simulink library "Vehicle_cl"  (R2020a)
settings: Solver=VariableStepAuto  StartTime=0.0  StopTime=10.0  RelTol=1e-3
undefined symbols (not defined in the file): CFN, EGR, ENG, ENV, ETM, FAN, IC, ICE, magnitude, RAD, TRAN, TSTAT, VEH, x_0
libraries: simulink_extras x2
settings Model: Creator=John Jr  LastModifiedBy=John Jr

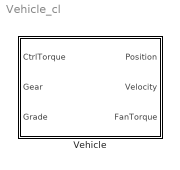
== system Vehicle_cl ==
  Vehicle : Subsystem

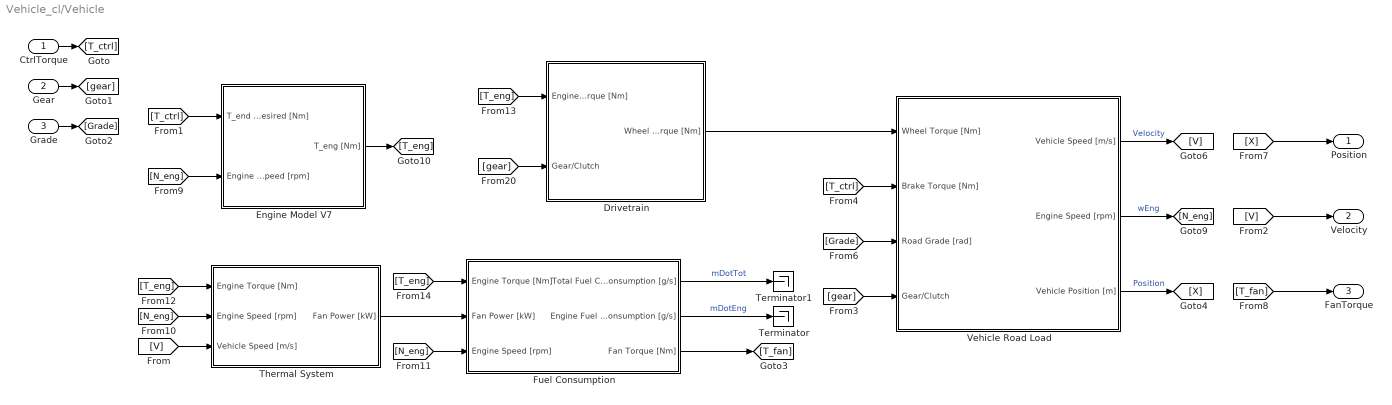
== system Vehicle_cl/Vehicle ==
  CtrlTorque : Inport
  Gear : Inport  Port=2
  Grade : Inport  Port=3
  Drivetrain : Subsystem
  Engine Model V7 : Subsystem
  Fuel Consumption : Subsystem
  Terminator : Terminator
  Terminator1 : Terminator
  Thermal System : Subsystem
  Vehicle Road Load : Subsystem
  Position : Outport
  Velocity : Outport  Port=2
  FanTorque : Outport  Port=3
  wires:
  [T_eng] -> Drivetrain/1(EngineTorque [Nm])
  Fuel Consumption/2(Engine Fuel Consumption [g/s]) -> Terminator/1  "mDotEng"
  [Grade] -> Vehicle Road Load/3(Road Grade [rad])
  [N_eng] -> Fuel Consumption/3(Engine Speed [rpm])
  Vehicle Road Load/3(Vehicle Position [m]) -> [X]  "Position"
  Fuel Consumption/3(Fan Torque [Nm]) -> [T_fan]
  Fuel Consumption/1(Total Fuel Consumption [g/s]) -> Terminator1/1  "mDotTot"
  Gear/1 -> [gear]
  Vehicle Road Load/2(Engine Speed [rpm]) -> [N_eng]  "wEng"
  [T_eng] -> Thermal System/1(Engine Torque [Nm])
  [T_ctrl] -> Vehicle Road Load/2(Brake Torque [Nm])
  [gear] -> Vehicle Road Load/4("Gear/Clutch ")
  [T_eng] -> Fuel Consumption/1(Engine Torque [Nm])
  [T_ctrl] -> Engine Model V7/1(T_end Desired [Nm])
  [gear] -> Drivetrain/2(Gear/Clutch)
  CtrlTorque/1 -> [T_ctrl]
  [N_eng] -> Engine Model V7/2(Engine Speed [rpm])
  Engine Model V7/1(T_eng [Nm]) -> [T_eng]
  [V] -> Thermal System/3(Vehicle Speed [m/s])
  Vehicle Road Load/1(Vehicle Speed [m/s]) -> [V]  "Velocity"
  Drivetrain/1(Wheel Torque [Nm]) -> Vehicle Road Load/1(Wheel Torque [Nm])
  [N_eng] -> Thermal System/2(Engine Speed [rpm])
  Thermal System/1(" Fan Power [kW]") -> Fuel Consumption/2(" Fan Power [kW]")
  Grade/1 -> [Grade]
  [T_fan] -> FanTorque/1
  [V] -> Velocity/1
  [X] -> Position/1

== system Vehicle_cl/Vehicle/Drivetrain ==
  EngineTorque [Nm] : Inport
  Gear/Clutch : Inport  Port=2
  Bus Selector : BusSelector  OutputSignals=Gear
  Gain2 : Gain  Gain=TRAN.finalDrive
  Gain3 : Gain  Gain=TRAN.gearEfficiency
  Gear Ratios : Lookup_n-D  NumberOfTableDimensions=1  BreakpointsForDimension1=[1:TRAN.numGears]  Table=TRAN.gears  ExtrapMethod=Clip  UseLastTableValue=on  InternalRulePriority=Speed  RndMeth=Simplest  InputSameDT=on
  Product1 : Product  Inputs=3
  Round : Rounding  Operator=round
  Transfe Fcn (with initial outputs) : simulink_extras/Additional Linear/Transfer Fcn (with initial outputs)  N=[1]  D="[.04 .4  1]"  Y0=0  U0=0
  Transmission Efficiency : Lookup_n-D  NumberOfTableDimensions=1  BreakpointsForDimension1=[1:TRAN.numGears]  Table=TRAN.transEfficiency  ExtrapMethod=Clip  UseLastTableValue=on  InternalRulePriority=Speed  RndMeth=Simplest  InputSameDT=on
  Wheel Torque [Nm] : Outport  VectorParamsAs1DForOutWhenUnconnected=off
  wires:
  Gear Ratios/1 -> Gain2/1
  Gain2/1 -> Product1/3
  Transmission Efficiency/1 -> Gain3/1
  Gain3/1 -> Product1/2
  Product1/1 -> Wheel Torque [Nm]/1  "whlTorque"
  EngineTorque [Nm]/1 -> Product1/1
  Transfe Fcn (with initial outputs)/1 -> Transmission Efficiency/1, Round/1
  Gear/Clutch/1 -> Bus Selector/1
  Bus Selector/1 -> Transfe Fcn (with initial outputs)/1  "<Gear>"
  Round/1 -> Gear Ratios/1

== system Vehicle_cl/Vehicle/Engine Model V7 ==
  T_end Desired [Nm] : Inport
  Engine Speed [rpm] : Inport  Port=2
  Bus Selector : BusSelector  OutputSignals=T_eng
  "Engine Breathing " : Subsystem
  Fuel Model : Subsystem
  Torque Production : Subsystem
  T_eng [Nm] : Outport  VectorParamsAs1DForOutWhenUnconnected=off
  wires:
  "Engine Breathing "/1(m_eng [kg/s]) -> Fuel Model/2(m_dot_eng [kg/s])
  Fuel Model/1(fuel [mg/cyc]) -> Torque Production/2(fuel [mg/cyc])
  Engine Speed [rpm]/1 -> "Engine Breathing "/1(Engine Speed [rpm]), Fuel Model/1(N [RPM]), Torque Production/1(N [RPM])
  Torque Production/1(T_eng [Nm]) -> T_eng [Nm]/1  "T_eng_act"
  T_end Desired [Nm]/1 -> Bus Selector/1
  Bus Selector/1 -> Torque Production/3(Engine Torqe Des [Nm]), Fuel Model/3(Engine Torqe Des [Nm]), "Engine Breathing "/2(Engine Torqe Des [Nm])  "<T_eng>"

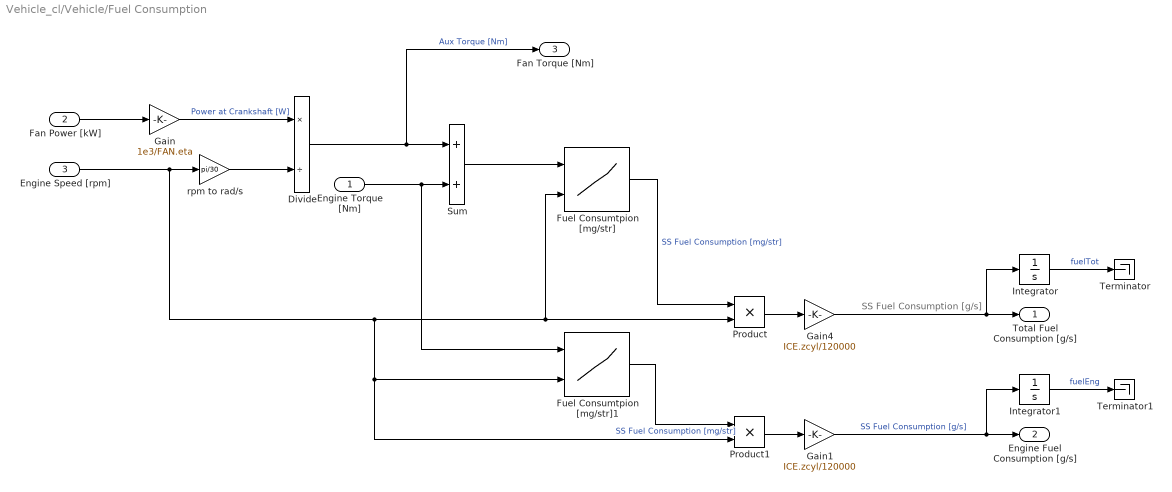
== system Vehicle_cl/Vehicle/Fuel Consumption ==
  note: SS Fuel Consumption [g/s]
  Engine Torque [Nm] : Inport
  " Fan Power [kW]" : Inport  Port=2
  Engine Speed [rpm] : Inport  Port=3
  Divide : Product  Inputs=*/
  Fuel Consumtpion [mg/str] : Lookup_n-D  BreakpointsForDimension1=ICE.FC.T  BreakpointsForDimension2=ICE.FC.N  Table=ICE.FC.mdot_mgpstr  InternalRulePriority=Speed  RndMeth=Simplest  InputSameDT=on
  Fuel Consumtpion [mg/str]1 : Lookup_n-D  BreakpointsForDimension1=ICE.FC.T  BreakpointsForDimension2=ICE.FC.N  Table=ICE.FC.mdot_mgpstr  InternalRulePriority=Speed  RndMeth=Simplest  InputSameDT=on
  Gain : Gain  Gain=1e3/FAN.eta
  Gain1 : Gain  Gain=ICE.zcyl/120000
  Gain4 : Gain  Gain=ICE.zcyl/120000
  Integrator : Integrator
  Integrator1 : Integrator
  Product : Product
  Product1 : Product
  Sum : Sum
  Terminator : Terminator
  Terminator1 : Terminator
  rpm to rad/s : Gain  Gain=pi/30
  Total Fuel Consumption [g/s] : Outport  VectorParamsAs1DForOutWhenUnconnected=off
  Engine Fuel Consumption [g/s] : Outport  Port=2  VectorParamsAs1DForOutWhenUnconnected=off
  Fan Torque [Nm] : Outport  Port=3  VectorParamsAs1DForOutWhenUnconnected=off
  wires:
  " Fan Power [kW]"/1 -> Gain/1
  Gain/1 -> Divide/1  "Power at Crankshaft [W]"
  rpm to rad/s/1 -> Divide/2
  Divide/1 -> Fan Torque [Nm]/1, Sum/1  "Aux Torque [Nm]"
  Gain4/1 -> Integrator/1, Total Fuel Consumption [g/s]/1
  Gain1/1 -> Integrator1/1, Engine Fuel Consumption [g/s]/1  "SS Fuel Consumption [g/s]"
  Fuel Consumtpion [mg/str]/1 -> Product/1  "SS Fuel Consumption [mg/str]"
  Product/1 -> Gain4/1
  Sum/1 -> Fuel Consumtpion [mg/str]/1
  Engine Speed [rpm]/1 -> Product1/2, Fuel Consumtpion [mg/str]1/2, Fuel Consumtpion [mg/str]/2, Product/2, rpm to rad/s/1
  Fuel Consumtpion [mg/str]1/1 -> Product1/1  "SS Fuel Consumption [mg/str]"
  Product1/1 -> Gain1/1
  Engine Torque [Nm]/1 -> Fuel Consumtpion [mg/str]1/1, Sum/2
  Integrator/1 -> Terminator/1  "fuelTot"
  Integrator1/1 -> Terminator1/1  "fuelEng"

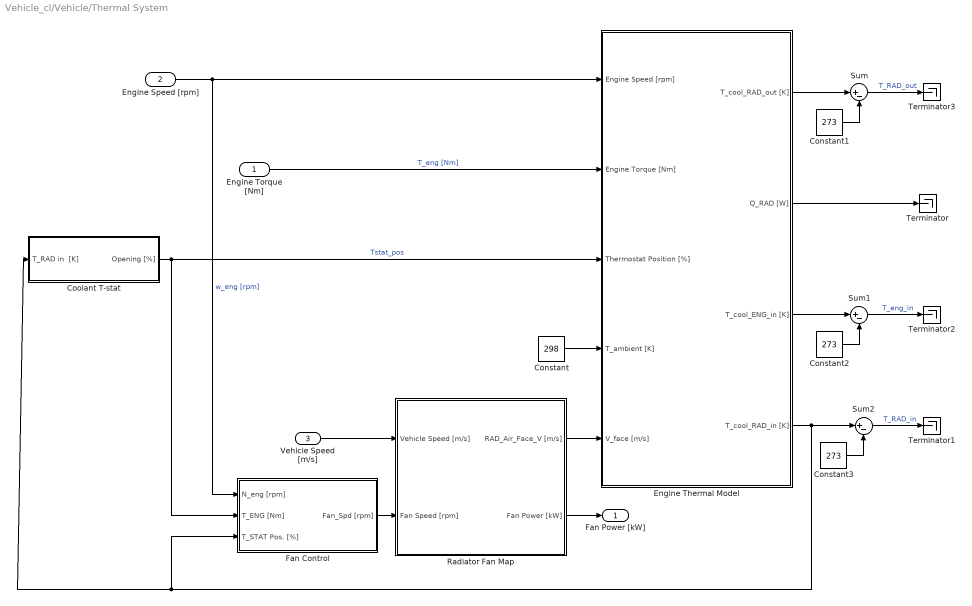
== system Vehicle_cl/Vehicle/Thermal System ==
  Engine Torque [Nm] : Inport
  Engine Speed [rpm] : Inport  Port=2
  Vehicle Speed [m/s] : Inport  Port=3
  Constant : Constant  Value=298
  Constant1 : Constant  Value=273
  Constant2 : Constant  Value=273
  Constant3 : Constant  Value=273
  Coolant T-stat : Subsystem
  Engine Thermal Model : Subsystem
  Fan Control : Subsystem
  Radiator Fan Map : Subsystem
  Sum : Sum  Inputs=|+-
  Sum1 : Sum  Inputs=|+-
  Sum2 : Sum  Inputs=|+-
  Terminator{,1..3} (4 alike) : Terminator
  " Fan Power [kW]" : Outport  VectorParamsAs1DForOutWhenUnconnected=off
  wires:
  Fan Control/1(Fan_Spd [rpm]) -> Radiator Fan Map/2(Fan Speed [rpm])
  Engine Speed [rpm]/1 -> Fan Control/1(N_eng [rpm]), Engine Thermal Model/1(Engine Speed [rpm])  "w_eng [rpm]"
  Radiator Fan Map/2(Fan Power [kW]) -> " Fan Power [kW]"/1
  Constant/1 -> Engine Thermal Model/4(T_ambient [K])
  Engine Torque [Nm]/1 -> Engine Thermal Model/2(Engine Torque [Nm])  "T_eng [Nm]"
  Radiator Fan Map/1(RAD_Air_Face_V [m/s]) -> Engine Thermal Model/5(V_face [m/s])
  Engine Thermal Model/1(T_cool_RAD_out [K]) -> Sum/1
  Constant1/1 -> Sum/2
  Sum/1 -> Terminator3/1  "T_RAD_out"
  Engine Thermal Model/3(T_cool_ENG_in [K]) -> Sum1/1
  Constant2/1 -> Sum1/2
  Sum1/1 -> Terminator2/1  "T_eng_in"
  Engine Thermal Model/4(T_cool_RAD_in [K]) -> Sum2/1, Fan Control/3(T_STAT Pos. [%]), Coolant T-stat/1(T_RAD in  [K])
  Constant3/1 -> Sum2/2
  Sum2/1 -> Terminator1/1  "T_RAD_in"
  Vehicle Speed [m/s]/1 -> Radiator Fan Map/1(Vehicle Speed [m/s])
  Engine Thermal Model/2(Q_RAD [W]) -> Terminator/1
  Coolant T-stat/1(Opening [%]) -> Fan Control/2(T_ENG [Nm]), Engine Thermal Model/3(Thermostat Position [%])  "Tstat_pos"

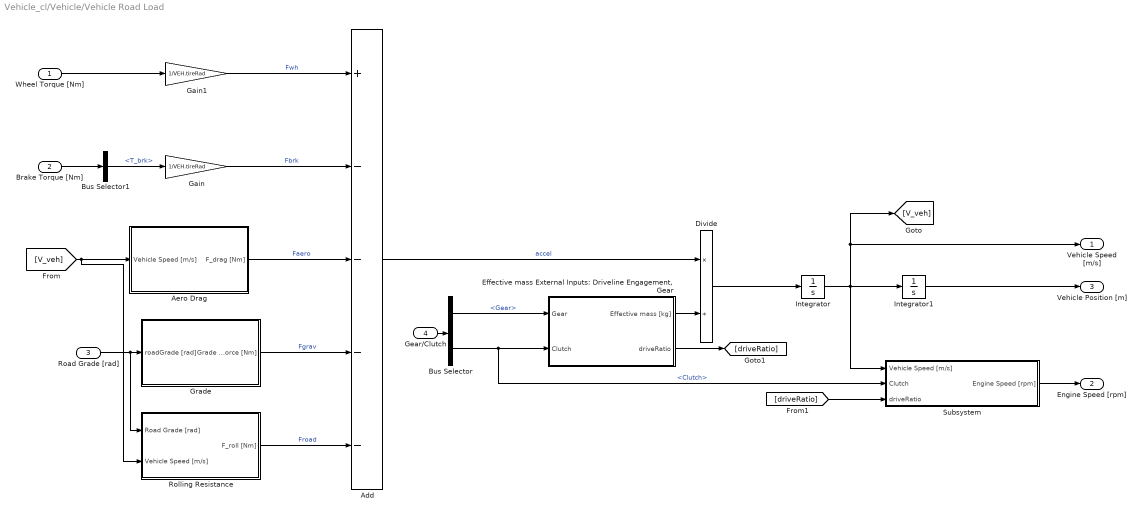
== system Vehicle_cl/Vehicle/Vehicle Road Load ==
  Wheel Torque [Nm] : Inport
  Brake Torque [Nm] : Inport  Port=2
  Road Grade [rad] : Inport  Port=3
  "Gear/Clutch " : Inport  Port=4
  Add : Sum  Inputs=+----
  Aero Drag : Subsystem
  Bus Selector : BusSelector  OutputSignals=Gear,Clutch
  Bus Selector1 : BusSelector  OutputSignals=T_brk
  Divide : Product  Inputs=*/
  "Effective mass External Inputs: Driveline Engagement, Gear" : Subsystem
  Gain : Gain  Gain=1/VEH.tireRad
  Gain1 : Gain  Gain=1/VEH.tireRad
  Grade : Subsystem
  Integrator : Integrator  LimitOutput=on  LowerSaturationLimit=0
  Integrator1 : Integrator  InitialCondition=x_0  LimitOutput=on  LowerSaturationLimit=0
  Rolling Resistance : Subsystem
  Subsystem : Subsystem
  Vehicle Speed [m/s] : Outport  VectorParamsAs1DForOutWhenUnconnected=off
  Engine Speed [rpm] : Outport  Port=2  VectorParamsAs1DForOutWhenUnconnected=off
  Vehicle Position [m] : Outport  Port=3  VectorParamsAs1DForOutWhenUnconnected=off
  wires:
  Integrator/1 -> Subsystem/1(Vehicle Speed [m/s]), Integrator1/1, Vehicle Speed [m/s]/1, [V_veh]
  Aero Drag/1(F_drag [Nm]) -> Add/3  "Faero"
  Grade/1(Grade Force [Nm]) -> Add/4  "Fgrav"
  Gain/1 -> Add/2  "Fbrk"
  Wheel Torque [Nm]/1 -> Gain1/1
  Gain1/1 -> Add/1  "Fwh"
  Rolling Resistance/1(F_roll [Nm]) -> Add/5  "Froad"
  Add/1 -> Divide/1  "accel"
  Divide/1 -> Integrator/1
  [V_veh] -> Aero Drag/1(Vehicle Speed [m/s]), Rolling Resistance/2(Vehicle Speed [m/s])
  Road Grade [rad]/1 -> Rolling Resistance/1(Road Grade [rad]), Grade/1(roadGrade [rad])
  Subsystem/1(Engine Speed [rpm]) -> Engine Speed [rpm]/1
  "Effective mass External Inputs: Driveline Engagement, Gear"/1("Effective mass [kg] ") -> Divide/2
  Integrator1/1 -> Vehicle Position [m]/1
  "Gear/Clutch "/1 -> Bus Selector/1
  Bus Selector/1 -> "Effective mass External Inputs: Driveline Engagement, Gear"/1(Gear)  "<Gear>"
  Bus Selector/2 -> Subsystem/2(Clutch), "Effective mass External Inputs: Driveline Engagement, Gear"/2(Clutch)  "<Clutch>"
  Brake Torque [Nm]/1 -> Bus Selector1/1
  Bus Selector1/1 -> Gain/1  "<T_brk>"
  "Effective mass External Inputs: Driveline Engagement, Gear"/2(driveRatio) -> [driveRatio]
  [driveRatio] -> Subsystem/3(driveRatio)

== system Vehicle_cl/Vehicle/Engine Model V7/Engine Breathing  ==
  Engine Speed [rpm] : Inport
  Engine Torqe Des [Nm] : Inport  Port=2
  Air Dynamics : Subsystem
  Engine Torqe Des [Nm]1 : InportShadow  Port=2
  Gain : Gain  Gain=1e3
  Gain1 : Gain  Gain=ICE.Vd/(120*ENV.R)
  Intake Manifold Pressure [kPa] : Lookup_n-D  BreakpointsForDimension1=ICE.air.Torque  BreakpointsForDimension2=ICE.air.N  Table=ICE.air.MAP  InternalRulePriority=Speed  RndMeth=Simplest  InputSameDT=on
  Intake Manifold Temperature [K] : Lookup_n-D  BreakpointsForDimension1=ICE.air.Torque  BreakpointsForDimension2=ICE.air.N  Table=ICE.air.MAT  InternalRulePriority=Speed  RndMeth=Simplest  InputSameDT=on
  Memory : Memory
  Model for VE : Subsystem
  Product : Product  Inputs=***/
  Subtract : Sum  Inputs=+-
  m_eng [kg/s] : Outport  VectorParamsAs1DForOutWhenUnconnected=off
  wires:
  Model for VE/1(VE [-]) -> Product/1
  Product/1 -> Gain1/1
  Gain1/1 -> Air Dynamics/1(m_dot_SS [kg/s])  "m_dot_SS"
  Intake Manifold Temperature [K]/1 -> Product/4, Model for VE/2(TIM [K])
  Engine Speed [rpm]/1 -> Intake Manifold Pressure [kPa]/2, Intake Manifold Temperature [K]/2, Product/3, Model for VE/3(N_eng [RPM])
  Engine Torqe Des [Nm]/1 -> Intake Manifold Temperature [K]/1, Intake Manifold Pressure [kPa]/1
  Gain/1 -> Product/2
  Intake Manifold Pressure [kPa]/1 -> Gain/1, Model for VE/1(MAP [kPa])
  Air Dynamics/1(m_dot_eng [kg/s]) -> m_eng [kg/s]/1  "m_dot_eng"
  Engine Torqe Des [Nm]1/1 -> Memory/1, Subtract/1
  Memory/1 -> Subtract/2
  Subtract/1 -> Air Dynamics/2(detla Torque [Nm])  "\\delta T Requested"

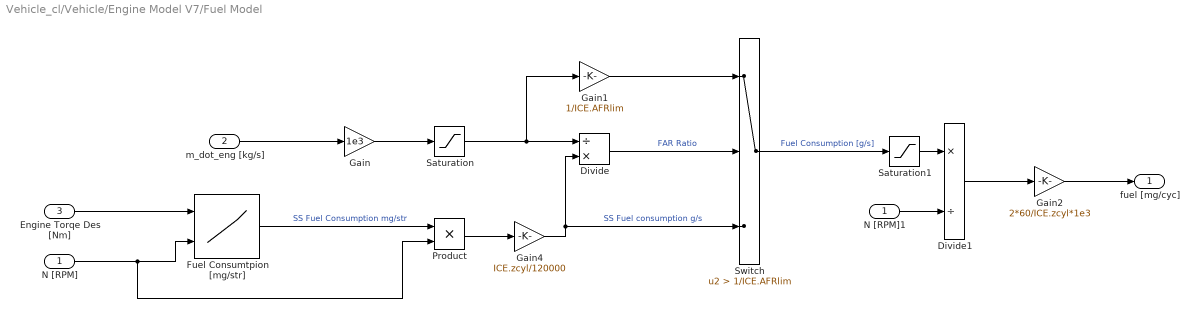
== system Vehicle_cl/Vehicle/Engine Model V7/Fuel Model ==
  N [RPM] : Inport
  m_dot_eng [kg/s] : Inport  Port=2
  Engine Torqe Des [Nm] : Inport  Port=3
  Divide : Product  Inputs=/*
  Divide1 : Product  Inputs=*/
  Fuel Consumtpion [mg/str] : Lookup_n-D  BreakpointsForDimension1=ICE.FC.T  BreakpointsForDimension2=ICE.FC.N  Table=ICE.FC.mdot_mgpstr  InternalRulePriority=Speed  RndMeth=Simplest  InputSameDT=on
  Gain : Gain  Gain=1e3
  Gain1 : Gain  Gain=1/ICE.AFRlim
  Gain2 : Gain  Gain=2*60/ICE.zcyl*1e3
  Gain4 : Gain  Gain=ICE.zcyl/120000
  N [RPM]1 : InportShadow
  Product : Product
  Saturation : Saturate  UpperLimit=inf  LowerLimit=0.001
  Saturation1 : Saturate  UpperLimit=inf  LowerLimit=0
  Switch : Switch  Criteria=u2 > Threshold  Threshold=1/ICE.AFRlim
  fuel [mg/cyc] : Outport  VectorParamsAs1DForOutWhenUnconnected=off
  wires:
  m_dot_eng [kg/s]/1 -> Gain/1
  N [RPM]/1 -> Product/2, Fuel Consumtpion [mg/str]/2
  Divide/1 -> Switch/2  "FAR Ratio"
  Fuel Consumtpion [mg/str]/1 -> Product/1  "SS Fuel Consumption mg/str"
  Gain/1 -> Saturation/1
  Gain1/1 -> Switch/1
  N [RPM]1/1 -> Divide1/2
  Divide1/1 -> Gain2/1
  Switch/1 -> Saturation1/1  "Fuel Consumption [g/s]"
  Saturation/1 -> Gain1/1, Divide/1
  Gain2/1 -> fuel [mg/cyc]/1
  Saturation1/1 -> Divide1/1
  Product/1 -> Gain4/1
  Gain4/1 -> Switch/3, Divide/2  "SS Fuel consumption g/s"
  Engine Torqe Des [Nm]/1 -> Fuel Consumtpion [mg/str]/1

== system Vehicle_cl/Vehicle/Engine Model V7/Torque Production ==
  N [RPM] : Inport
  fuel [mg/cyc] : Inport  Port=2
  Engine Torqe Des [Nm] : Inport  Port=3
  Add : Sum  Inputs=+--
  Constant : Constant  Value=0
  Constant1 : Constant  Value=40/ICE.Vd*(4*pi)
  FMEP Model : Lookup_n-D  BreakpointsForDimension1=ICE.FMEP.RPM_vec  BreakpointsForDimension2=ICE.FMEP.fuel_vec  Table=ICE.FMEP.FMEP_surf  InternalRulePriority=Speed  RndMeth=Simplest  InputSameDT=on
  Fuel Dynamics : Subsystem
  Gain1 : Gain  Gain=ICE.Vd/(4*pi)
  IMEP Model : Lookup_n-D  BreakpointsForDimension1=ICE.IMEP.N  BreakpointsForDimension2=ICE.IMEP.m_fuel  Table=ICE.IMEP.IMEP'  UseLastTableValue=on  InternalRulePriority=Speed  RndMeth=Simplest  InputSameDT=on
  Memory : Memory
  Subtract : Sum  Inputs=+-
  Switch : Switch  Criteria=u2 > Threshold
  T_eng [Nm] : Outport  VectorParamsAs1DForOutWhenUnconnected=off
  wires:
  FMEP Model/1 -> Add/2  "FMEP [Pa]"
  IMEP Model/1 -> Add/1  "IMEP [Pa]"
  Add/1 -> Gain1/1  "BMEP [Pa]"
  N [RPM]/1 -> IMEP Model/1, FMEP Model/1
  fuel [mg/cyc]/1 -> IMEP Model/2, Switch/2, FMEP Model/2
  Gain1/1 -> Fuel Dynamics/1(T_SS [Nm])
  Engine Torqe Des [Nm]/1 -> Memory/1, Subtract/1
  Memory/1 -> Subtract/2
  Subtract/1 -> Fuel Dynamics/2(detla Torque [Nm])  "\\delta T Requested"
  Fuel Dynamics/1(Torque [Nm]) -> T_eng [Nm]/1
  Switch/1 -> Add/3
  Constant/1 -> Switch/1
  Constant1/1 -> Switch/3

== system Vehicle_cl/Vehicle/Thermal System/Coolant T-stat ==
  T_RAD in  [K] : Inport
  Add : Sum
  Constant : Constant  Value=TSTAT.tau
  Divide : Product  Inputs=*/
  Fcn1 : Fcn  Expr=u-273
  Gain : Gain  Gain=0.85
  Gain1 : Gain  Gain=0.15
  Integrator : Integrator  InitialCondition=TSTAT.IC
  Sum : Sum  Inputs=+-
  Temp - Mechanical Closing : Lookup  InputValues=TSTAT.mclosing(:,1)  Table=TSTAT.mclosing(:,2)  LookUpMeth=Interpolation-Use End Values
  Temp - Mechanical Opening : Lookup  InputValues=TSTAT.mopening(:,1)  Table=TSTAT.mopening(:,2)  LookUpMeth=Interpolation-Use End Values
  Opening [%] : Outport  VectorParamsAs1DForOutWhenUnconnected=off
  wires:
  Temp - Mechanical Opening/1 -> Gain/1
  Temp - Mechanical Closing/1 -> Gain1/1
  Add/1 -> Sum/1
  Sum/1 -> Divide/1
  Constant/1 -> Divide/2
  Divide/1 -> Integrator/1
  Integrator/1 -> Sum/2, Opening [%]/1
  T_RAD in  [K]/1 -> Fcn1/1
  Gain/1 -> Add/1
  Gain1/1 -> Add/2
  Fcn1/1 -> Temp - Mechanical Opening/1, Temp - Mechanical Closing/1

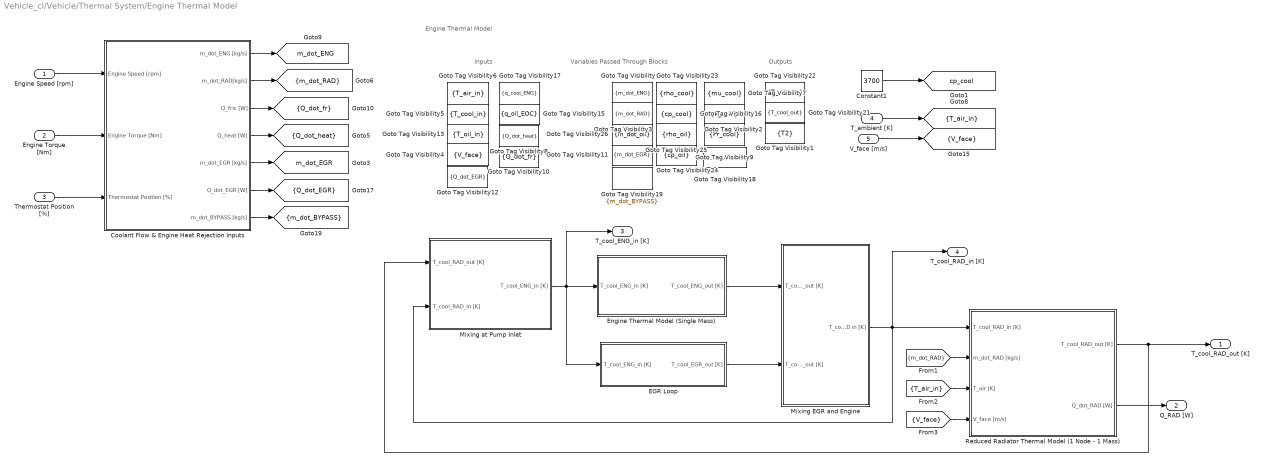
== system Vehicle_cl/Vehicle/Thermal System/Engine Thermal Model ==
  note: Variables Passed Through Blocks
  note: Inputs
  note: Engine Thermal Model
  note: Outputs
  Engine Speed [rpm] : Inport
  Engine Torque [Nm] : Inport  Port=2
  Thermostat Position [%] : Inport  Port=3
  T_ambient [K] : Inport  Port=4
  V_face [m/s] : Inport  Port=5
  Constant1 : Constant  Value=3700
  Coolant Flow & Engine Heat Rejection Inputs : Subsystem
      mask DialogControl DescGroupVar Prompt: Coolant Flow Rate And Engine Heat Rejection Inputs
  EGR Loop : Subsystem
  Engine Thermal Model (Single Mass) : Subsystem
  Goto Tag Visibility1 : GotoTagVisibility  GotoTag=T2
  Goto Tag Visibility10 : GotoTagVisibility  GotoTag=Q_dot_fr
  Goto Tag Visibility11 : GotoTagVisibility  GotoTag=m_dot_EGR
  Goto Tag Visibility12 : GotoTagVisibility  GotoTag=Q_dot_EGR
  Goto Tag Visibility13 : GotoTagVisibility  GotoTag=T_oil_in
  Goto Tag Visibility14 : GotoTagVisibility  GotoTag=m_dot_ENG
  Goto Tag Visibility15 : GotoTagVisibility  GotoTag=q_oil_EOC
  Goto Tag Visibility16 : GotoTagVisibility  GotoTag=cp_cool
  Goto Tag Visibility17 : GotoTagVisibility  GotoTag=q_cool_ENG
  Goto Tag Visibility18 : GotoTagVisibility  GotoTag=T_cool_ENG_out
  Goto Tag Visibility19 : GotoTagVisibility  GotoTag=m_dot_BYPASS
  Goto Tag Visibility2 : GotoTagVisibility  GotoTag=k_cool
  Goto Tag Visibility21 : GotoTagVisibility  GotoTag=T_cool_out
  Goto Tag Visibility22 : GotoTagVisibility  GotoTag=T_oil_out
  Goto Tag Visibility23 : GotoTagVisibility  GotoTag=rho_cool
  Goto Tag Visibility24 : GotoTagVisibility  GotoTag=cp_oil
  Goto Tag Visibility25 : GotoTagVisibility  GotoTag=rho_oil
  Goto Tag Visibility26 : GotoTagVisibility  GotoTag=m_dot_oil
  Goto Tag Visibility3 : GotoTagVisibility  GotoTag=m_dot_RAD
  Goto Tag Visibility4 : GotoTagVisibility  GotoTag=V_face
  Goto Tag Visibility5 : GotoTagVisibility  GotoTag=T_cool_in
  Goto Tag Visibility6 : GotoTagVisibility  GotoTag=T_air_in
  Goto Tag Visibility7 : GotoTagVisibility  GotoTag=mu_cool
  Goto Tag Visibility8 : GotoTagVisibility  GotoTag=Q_dot_heat
  Goto Tag Visibility9 : GotoTagVisibility  GotoTag=Pr_cool
  Mixing EGR and Engine : Subsystem
  "Mixing at Pump Inlet " : Subsystem
  Reduced Radiator Thermal Model (1 Node - 1 Mass) : Subsystem
  T_cool_RAD_out [K] : Outport  VectorParamsAs1DForOutWhenUnconnected=off
  Q_RAD [W] : Outport  Port=2  VectorParamsAs1DForOutWhenUnconnected=off
  T_cool_ENG_in [K] : Outport  Port=3  VectorParamsAs1DForOutWhenUnconnected=off
  T_cool_RAD_in [K] : Outport  Port=4  VectorParamsAs1DForOutWhenUnconnected=off
  tag scope: Q_dot_EGR=scoped, Q_dot_fr=scoped, Q_dot_heat=scoped, T_air_in=scoped, V_face=scoped, cp_cool=global, m_dot_BYPASS=scoped, m_dot_EGR=global, m_dot_ENG=global, m_dot_RAD=scoped
  wires:
  T_ambient [K]/1 -> [T_air_in]
  [m_dot_RAD] -> Reduced Radiator Thermal Model (1 Node - 1 Mass)/2(m_dot_RAD [kg/s])
  [T_air_in] -> Reduced Radiator Thermal Model (1 Node - 1 Mass)/3(T_air [K])
  V_face [m/s]/1 -> [V_face]
  [V_face] -> Reduced Radiator Thermal Model (1 Node - 1 Mass)/4(V_face [m/s])
  Reduced Radiator Thermal Model (1 Node - 1 Mass)/2(Q_dot_RAD [W]) -> Q_RAD [W]/1
  Reduced Radiator Thermal Model (1 Node - 1 Mass)/1(T_cool_RAD_out [K]) -> "Mixing at Pump Inlet "/1(T_cool_RAD_out [K]), T_cool_RAD_out [K]/1
  Constant1/1 -> [cp_cool]
  Coolant Flow & Engine Heat Rejection Inputs/5(m_dot_EGR [kg/s]) -> [m_dot_EGR]
  Coolant Flow & Engine Heat Rejection Inputs/6(Q_dot_EGR [W]) -> [Q_dot_EGR]
  Coolant Flow & Engine Heat Rejection Inputs/1(m_dot_ENG [kg/s]) -> [m_dot_ENG]
  Coolant Flow & Engine Heat Rejection Inputs/4(Q_heat [W]) -> [Q_dot_heat]
  Coolant Flow & Engine Heat Rejection Inputs/2(m_dot_RAD[kg/s]) -> [m_dot_RAD]
  Engine Torque [Nm]/1 -> Coolant Flow & Engine Heat Rejection Inputs/2(Engine Torque [Nm])
  Coolant Flow & Engine Heat Rejection Inputs/3(Q_fric [W]) -> [Q_dot_fr]
  Thermostat Position [%]/1 -> Coolant Flow & Engine Heat Rejection Inputs/3(Thermostat Position [%])
  Coolant Flow & Engine Heat Rejection Inputs/7(m_dot_BYPASS [kg/s]) -> [m_dot_BYPASS]
  Engine Speed [rpm]/1 -> Coolant Flow & Engine Heat Rejection Inputs/1(Engine Speed [rpm])
  Engine Thermal Model (Single Mass)/1(T_cool_ENG_out [K]) -> Mixing EGR and Engine/1(T_cool_ENG_out [K])
  EGR Loop/1(T_cool_EGR_out [K]) -> Mixing EGR and Engine/2(T_cool_EGR_out [K])
  Mixing EGR and Engine/1(T_cool_RAD in [K]) -> "Mixing at Pump Inlet "/2(T_cool_RAD_in [K]), Reduced Radiator Thermal Model (1 Node - 1 Mass)/1(T_cool_RAD_in [K]), T_cool_RAD_in [K]/1
  "Mixing at Pump Inlet "/1(T_cool_ENG_in [K]) -> T_cool_ENG_in [K]/1, Engine Thermal Model (Single Mass)/1(T_cool_ENG_in [K]), EGR Loop/1(T_cool_ENG_in [K])

== system Vehicle_cl/Vehicle/Thermal System/Fan Control ==
  note: Fan Controller
  N_eng [rpm] : Inport
  T_ENG [Nm] : Inport  Port=2
  T_STAT Pos. [%] : Inport  Port=3
  Fan Min Speed [rpm] : Constant  Value=200
  Fan OFF : Constant  Value=0
  "Fan ON " : Constant
  Fan Pulley Ratio : Constant  Value=FAN.pulley_ratio
  "IF T_eng is > 367 K and T_stat = 100% open, then Fan ON1" : Switch  Threshold=1
  Logical Operator1 : Logic  AllPortsSameDT=off  OutDataTypeStr=boolean
  Product2 : Product  Inputs=3
  Relay2 : Relay  OnSwitchValue=5  OffSwitchValue=0  OnOutputValue=0  OffOutputValue=1
  Relay3 : Relay  OnSwitchValue=25  OffSwitchValue=20
  Switch1 : Switch  Criteria=u2 > Threshold
  Fan_Spd [rpm] : Outport  VectorParamsAs1DForOutWhenUnconnected=off
  wires:
  Product2/1 -> Switch1/1, Switch1/2
  Relay2/1 -> Logical Operator1/2
  Fan Pulley Ratio/1 -> Product2/1
  T_STAT Pos. [%]/1 -> Relay3/1
  N_eng [rpm]/1 -> Product2/3
  Fan Min Speed [rpm]/1 -> Switch1/3
  Relay3/1 -> Logical Operator1/1
  Logical Operator1/1 -> "IF T_eng is > 367 K and T_stat = 100% open, then Fan ON1"/2
  T_ENG [Nm]/1 -> Relay2/1
  Fan OFF/1 -> "IF T_eng is > 367 K and T_stat = 100% open, then Fan ON1"/3
  "IF T_eng is > 367 K and T_stat = 100% open, then Fan ON1"/1 -> Product2/2
  "Fan ON "/1 -> "IF T_eng is > 367 K and T_stat = 100% open, then Fan ON1"/1
  Switch1/1 -> Fan_Spd [rpm]/1  "fanSpeed"

== system Vehicle_cl/Vehicle/Thermal System/Radiator Fan Map ==
  Vehicle Speed [m/s] : Inport
  Fan Speed [rpm] : Inport  Port=2
  Air Density : Constant  Value=RAD.Air_rho
  Divide : Product  Inputs=*//
  Face Area [m^2] : Constant  Value=RAD.A_face
  Fan Power Consumption [kW] : Lookup_n-D  NumberOfTableDimensions=1  BreakpointsForDimension1=FAN.Speed  Table=FAN.Power  RndMeth=Simplest  InputSameDT=on
  Fan Table : Lookup_n-D  BreakpointsForDimension1=FAN.N  BreakpointsForDimension2=FAN.Vspd  Table=FAN.RAD_AGS_o  ExtrapMethod=Clip  RndMeth=Simplest  InputSameDT=on
  RAD_Air_Face_V [m/s] : Outport  VectorParamsAs1DForOutWhenUnconnected=off
  Fan Power [kW] : Outport  Port=2  VectorParamsAs1DForOutWhenUnconnected=off
  wires:
  Fan Speed [rpm]/1 -> Fan Table/1, Fan Power Consumption [kW]/1
  Fan Table/1 -> Divide/1  "Rad_Air_Face_mdot [kg/s]"
  Divide/1 -> RAD_Air_Face_V [m/s]/1
  Air Density/1 -> Divide/3
  Vehicle Speed [m/s]/1 -> Fan Table/2
  Face Area [m^2]/1 -> Divide/2
  Fan Power Consumption [kW]/1 -> Fan Power [kW]/1

== system Vehicle_cl/Vehicle/Vehicle Road Load/Aero Drag ==
  Vehicle Speed [m/s] : Inport
  Gain1 : Gain  Gain=0.5*VEH.Af*ENV.rhoAir
  Math Function : Math  Operator=magnitude^2  SignedPower=on  SaturateOnIntegerOverflow=on
  Product : Product
  air drag coefficient3 : Constant  Value=VEH.Cd
  F_drag [Nm] : Outport  VectorParamsAs1DForOutWhenUnconnected=off
  wires:
  Vehicle Speed [m/s]/1 -> Math Function/1
  Gain1/1 -> F_drag [Nm]/1  "Drag"
  Math Function/1 -> Product/1
  air drag coefficient3/1 -> Product/2
  Product/1 -> Gain1/1

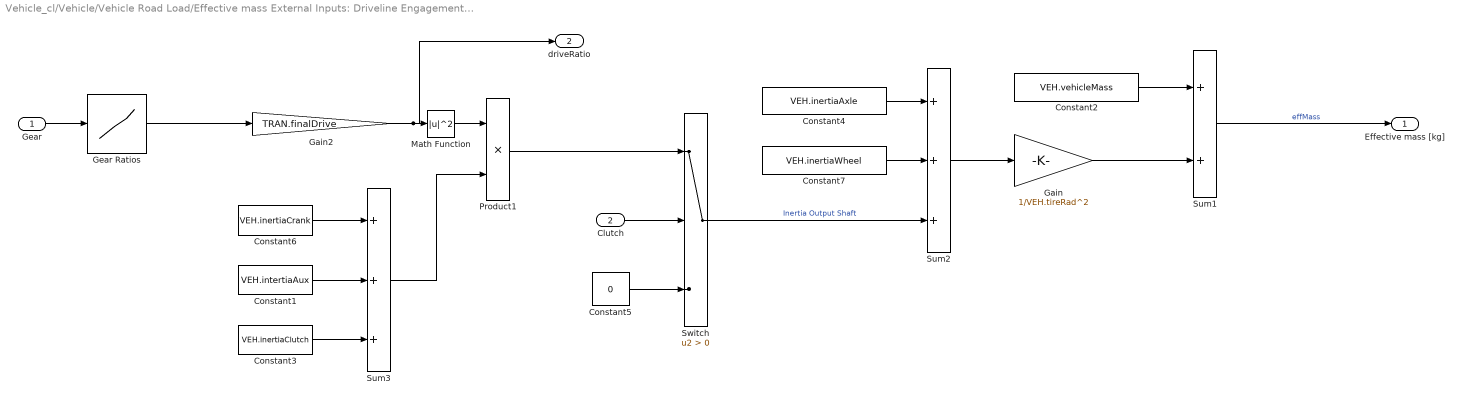
== system Vehicle_cl/Vehicle/Vehicle Road Load/Effective mass External Inputs: Driveline Engagement, Gear ==
  Gear : Inport
  Clutch : Inport  Port=2
  Constant1 : Constant  Value=VEH.intertiaAux
  Constant2 : Constant  Value=VEH.vehicleMass
  Constant3 : Constant  Value=VEH.inertiaClutch
  Constant4 : Constant  Value=VEH.inertiaAxle
  Constant5 : Constant  Value=0
  Constant6 : Constant  Value=VEH.inertiaCrank
  Constant7 : Constant  Value=VEH.inertiaWheel
  Gain : Gain  Gain=1/VEH.tireRad^2
  Gain2 : Gain  Gain=TRAN.finalDrive
  Gear Ratios : Lookup_n-D  NumberOfTableDimensions=1  BreakpointsForDimension1=[1:TRAN.numGears]  Table=TRAN.gears  ExtrapMethod=Clip  UseLastTableValue=on  InternalRulePriority=Speed  RndMeth=Simplest  InputSameDT=on
  Math Function : Math  Operator=magnitude^2  SignedPower=on  SaturateOnIntegerOverflow=on
  Product1 : Product
  Sum1 : Sum
  Sum2 : Sum  Inputs=+++
  Sum3 : Sum  Inputs=+++
  Switch : Switch  Criteria=u2 > Threshold
  "Effective mass [kg] " : Outport  VectorParamsAs1DForOutWhenUnconnected=off
  driveRatio : Outport  Port=2
  wires:
  Clutch/1 -> Switch/2
  Product1/1 -> Switch/1
  Constant5/1 -> Switch/3
  Switch/1 -> Sum2/3  "Inertia Output Shaft"
  Gear/1 -> Gear Ratios/1
  Gain2/1 -> driveRatio/1, Math Function/1
  Constant2/1 -> Sum1/1
  Gain/1 -> Sum1/2
  Sum2/1 -> Gain/1
  Constant4/1 -> Sum2/1
  Constant7/1 -> Sum2/2
  Constant6/1 -> Sum3/1
  Constant1/1 -> Sum3/2
  Constant3/1 -> Sum3/3
  Math Function/1 -> Product1/1
  Sum3/1 -> Product1/2
  Gear Ratios/1 -> Gain2/1
  Sum1/1 -> "Effective mass [kg] "/1  "effMass"

== system Vehicle_cl/Vehicle/Vehicle Road Load/Grade ==
  roadGrade [rad] : Inport
  Gain : Gain  Gain=VEH.vehicleMass*ENV.g
  Trigonometric Function1 : Trigonometry
  Grade Force [Nm] : Outport  VectorParamsAs1DForOutWhenUnconnected=off
  wires:
  Gain/1 -> Grade Force [Nm]/1
  Trigonometric Function1/1 -> Gain/1
  roadGrade [rad]/1 -> Trigonometric Function1/1

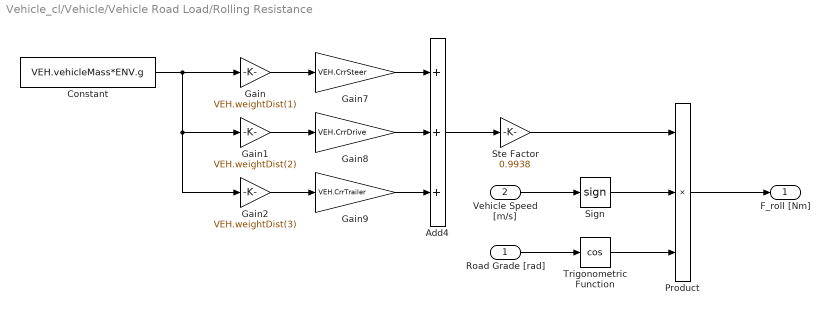
== system Vehicle_cl/Vehicle/Vehicle Road Load/Rolling Resistance ==
  Road Grade [rad] : Inport
  Vehicle Speed [m/s] : Inport  Port=2
  Add4 : Sum  Inputs=+++
  Constant : Constant  Value=VEH.vehicleMass*ENV.g
  Gain : Gain  Gain=VEH.weightDist(1)
  Gain1 : Gain  Gain=VEH.weightDist(2)
  Gain2 : Gain  Gain=VEH.weightDist(3)
  Gain7 : Gain  Gain=VEH.CrrSteer
  Gain8 : Gain  Gain=VEH.CrrDrive
  Gain9 : Gain  Gain=VEH.CrrTrailer
  Product : Product  Inputs=3
  Sign : Signum
  Ste Factor : Gain  Gain=0.9938
  Trigonometric Function : Trigonometry  Operator=cos
  F_roll [Nm] : Outport  VectorParamsAs1DForOutWhenUnconnected=off
  wires:
  Gain7/1 -> Add4/1
  Gain8/1 -> Add4/2
  Gain9/1 -> Add4/3
  Add4/1 -> Ste Factor/1
  Vehicle Speed [m/s]/1 -> Sign/1
  Product/1 -> F_roll [Nm]/1
  Constant/1 -> Gain2/1, Gain1/1, Gain/1
  Gain/1 -> Gain7/1
  Gain1/1 -> Gain8/1
  Gain2/1 -> Gain9/1
  Sign/1 -> Product/2
  Road Grade [rad]/1 -> Trigonometric Function/1
  Trigonometric Function/1 -> Product/3
  Ste Factor/1 -> Product/1

== system Vehicle_cl/Vehicle/Vehicle Road Load/Subsystem ==
  Vehicle Speed [m/s] : Inport
  Clutch : Inport  Port=2
  driveRatio : Inport  Port=3
  Constant1 : Constant  Value=-300
  Constant3 : Constant  Value=ICE.Nmin
  Disengaged : Subsystem  TreatAsAtomicUnit=on
  Engaged : Subsystem  TreatAsAtomicUnit=on
  Logical Operator : Logic  Operator=NOT  AllPortsSameDT=off  OutDataTypeStr=boolean
  Memory : Memory  InitialCondition=ICE.Nmin
  MinMax : MinMax  Function=max  Inputs=2
  Switch1 : Switch  Criteria=u2 > Threshold
  Engine Speed [rpm] : Outport  VectorParamsAs1DForOutWhenUnconnected=off
  wires:
  Clutch/1 -> Engaged/Enable, Logical Operator/1
  Disengaged/1(Out1) -> Switch1/1
  Constant1/1 -> Disengaged/2(T_eng)
  Logical Operator/1 -> Switch1/2, Disengaged/Enable
  Vehicle Speed [m/s]/1 -> Engaged/1(Vehicle Speed [m/s])
  driveRatio/1 -> Engaged/2(drive ratio)
  MinMax/1 -> Memory/1, Engine Speed [rpm]/1
  Switch1/1 -> MinMax/1
  Constant3/1 -> MinMax/2
  Memory/1 -> Disengaged/1(RPM init)
  Engaged/1(Out1) -> Switch1/3

== system Vehicle_cl/Vehicle/Engine Model V7/Engine Breathing /Air Dynamics ==
  m_dot_SS [kg/s] : Inport
  detla Torque [Nm] : Inport  Port=2
  Constant : Constant  Value=ICE.air_Tau_p
  Constant1 : Constant  Value=ICE.air_Tau_n
  Integrator : Integrator  InitialCondition=IC.mdot_eng
  Product : Product  Inputs=*/
  Subtract : Sum  Inputs=+-
  Switch : Switch  Criteria=u2 > Threshold
  m_dot_eng [kg/s] : Outport  VectorParamsAs1DForOutWhenUnconnected=off
  wires:
  m_dot_SS [kg/s]/1 -> Subtract/1
  detla Torque [Nm]/1 -> Switch/2
  Constant/1 -> Switch/1
  Constant1/1 -> Switch/3
  Integrator/1 -> Subtract/2, m_dot_eng [kg/s]/1
  Switch/1 -> [TauAir]
  Subtract/1 -> Product/1
  [TauAir] -> Product/2
  Product/1 -> Integrator/1

== system Vehicle_cl/Vehicle/Engine Model V7/Engine Breathing /Model for VE ==
  MAP [kPa] : Inport
  TIM [K] : Inport  Port=2
  N_eng [RPM] : Inport  Port=3
  Add2 : Sum
  Divide2 : Product  Inputs=*/*
  Function for the k1 coeff : Fcn  Expr=ICE.air.Q1(1)*u^ICE.air.Q1(2)+ICE.air.Q1(3)
  Function for the k1 coeff1 : Fcn  Expr=ICE.air.Q2(1)*u^2+ICE.air.Q2(2)*u+ICE.air.Q2(3)
  kPa to Pa : Gain  Gain=1e3
  VE [-] : Outport  VectorParamsAs1DForOutWhenUnconnected=off
  wires:
  N_eng [RPM]/1 -> Function for the k1 coeff1/1, Function for the k1 coeff/1
  Function for the k1 coeff/1 -> Add2/1  "k1 [-]"
  Function for the k1 coeff1/1 -> Divide2/1  "k2 [-]"
  MAP [kPa]/1 -> kPa to Pa/1
  TIM [K]/1 -> Divide2/3
  Divide2/1 -> Add2/2
  Add2/1 -> VE [-]/1
  kPa to Pa/1 -> Divide2/2

== system Vehicle_cl/Vehicle/Engine Model V7/Torque Production/Fuel Dynamics ==
  T_SS [Nm] : Inport
  detla Torque [Nm] : Inport  Port=2
  Constant : Constant  Value=ICE.fuel_Tau_p
  Constant1 : Constant  Value=ICE.fuel_Tau_n
  Integrator : Integrator  InitialCondition=IC.mdot_eng
  Product : Product  Inputs=*/
  Subtract : Sum  Inputs=+-
  Switch : Switch  Criteria=u2 > Threshold
  Torque [Nm] : Outport  VectorParamsAs1DForOutWhenUnconnected=off
  wires:
  T_SS [Nm]/1 -> Subtract/1
  detla Torque [Nm]/1 -> Switch/2
  Constant/1 -> Switch/1
  Constant1/1 -> Switch/3
  Integrator/1 -> Subtract/2, Torque [Nm]/1
  Switch/1 -> [TauFuel]
  Subtract/1 -> Product/1
  [TauFuel] -> Product/2
  Product/1 -> Integrator/1

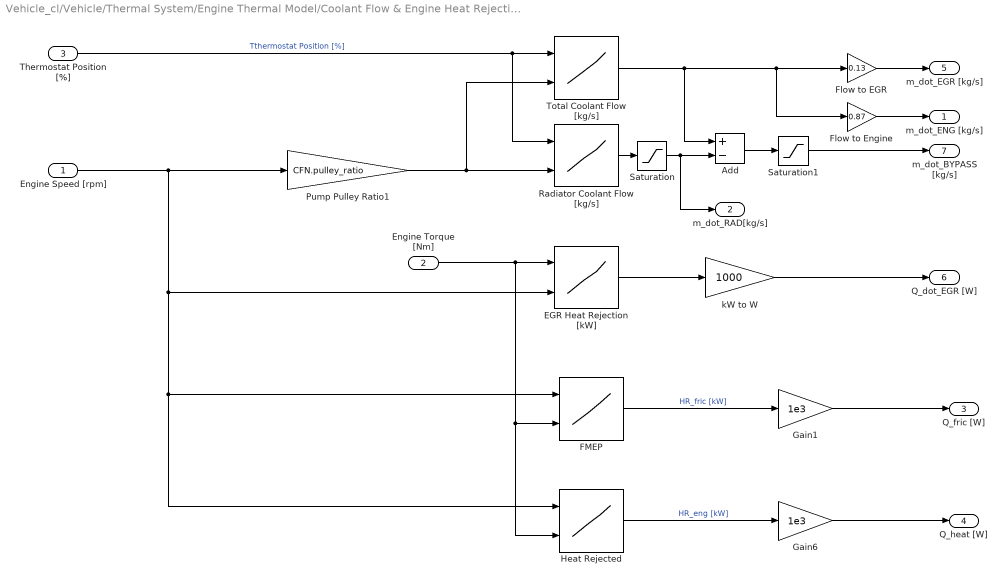
== system Vehicle_cl/Vehicle/Thermal System/Engine Thermal Model/Coolant Flow & Engine Heat Rejection Inputs ==
  Engine Speed [rpm] : Inport
  Engine Torque [Nm] : Inport  Port=2
  Thermostat Position [%] : Inport  Port=3
  Add : Sum  Inputs=+-
  EGR Heat Rejection [kW] : Lookup_n-D  BreakpointsForDimension1=EGR.Tau_Eng  BreakpointsForDimension2=EGR.Omega_Eng  Table=EGR.table_Heat_Transfered  ExtrapMethod=Clip  InternalRulePriority=Speed  RndMeth=Simplest  InputSameDT=on
  FMEP : Lookup_n-D  BreakpointsForDimension1=ENG.N  BreakpointsForDimension2=ENG.T  Table=ENG.FMEP  ExtrapMethod=Clip  RndMeth=Simplest  InputSameDT=on
  Flow to EGR : Gain  Gain=0.13
  Flow to Engine : Gain  Gain=0.87
  Gain1 : Gain  Gain=1e3
  Gain6 : Gain  Gain=1e3
  Heat Rejected : Lookup_n-D  BreakpointsForDimension1=ENG.N  BreakpointsForDimension2=ENG.T  Table=ENG.HR  ExtrapMethod=Clip  RndMeth=Simplest  InputSameDT=on
  Pump Pulley Ratio1 : Gain  Gain=CFN.pulley_ratio
  Radiator Coolant Flow [kg/s] : Lookup_n-D  BreakpointsForDimension1=CFN.table_ITW_pos  BreakpointsForDimension2=CFN.table_pump_speed  Table=CFN.table_RAD_flow_rates  ExtrapMethod=Clip  InternalRulePriority=Speed  RndMeth=Simplest  InputSameDT=on
  Saturation : Saturate  UpperLimit=inf  LowerLimit=0  ZeroCross=off
  Saturation1 : Saturate  UpperLimit=inf  LowerLimit=0  ZeroCross=off
  Total Coolant Flow [kg/s] : Lookup_n-D  BreakpointsForDimension1=CFN.table_ITW_pos  BreakpointsForDimension2=CFN.table_pump_speed  Table=CFN.table_TOT_flow_rates  ExtrapMethod=Clip  InternalRulePriority=Speed  RndMeth=Simplest  InputSameDT=on
  kW to W : Gain  Gain=1000
  m_dot_ENG [kg/s] : Outport  VectorParamsAs1DForOutWhenUnconnected=off
  m_dot_RAD[kg/s] : Outport  Port=2  VectorParamsAs1DForOutWhenUnconnected=off
  Q_fric [W] : Outport  Port=3  VectorParamsAs1DForOutWhenUnconnected=off
  Q_heat [W] : Outport  Port=4  VectorParamsAs1DForOutWhenUnconnected=off
  m_dot_EGR [kg/s] : Outport  Port=5  VectorParamsAs1DForOutWhenUnconnected=off
  Q_dot_EGR [W] : Outport  Port=6  VectorParamsAs1DForOutWhenUnconnected=off
  m_dot_BYPASS [kg/s] : Outport  Port=7  VectorParamsAs1DForOutWhenUnconnected=off
  wires:
  Engine Speed [rpm]/1 -> Pump Pulley Ratio1/1, EGR Heat Rejection [kW]/2, FMEP/1, Heat Rejected/1
  FMEP/1 -> Gain1/1  "HR_fric [kW]"
  Heat Rejected/1 -> Gain6/1  "HR_eng [kW]"
  Thermostat Position [%]/1 -> Radiator Coolant Flow [kg/s]/1, Total Coolant Flow [kg/s]/1  "Tthermostat Position [%]"
  Flow to EGR/1 -> m_dot_EGR [kg/s]/1
  Flow to Engine/1 -> m_dot_ENG [kg/s]/1
  EGR Heat Rejection [kW]/1 -> kW to W/1
  kW to W/1 -> Q_dot_EGR [W]/1
  Pump Pulley Ratio1/1 -> Total Coolant Flow [kg/s]/2, Radiator Coolant Flow [kg/s]/2
  Radiator Coolant Flow [kg/s]/1 -> Saturation/1
  Engine Torque [Nm]/1 -> Heat Rejected/2, FMEP/2, EGR Heat Rejection [kW]/1
  Total Coolant Flow [kg/s]/1 -> Add/1, Flow to Engine/1, Flow to EGR/1
  Saturation/1 -> m_dot_RAD[kg/s]/1, Add/2
  Add/1 -> Saturation1/1
  Saturation1/1 -> m_dot_BYPASS [kg/s]/1
  Gain1/1 -> Q_fric [W]/1
  Gain6/1 -> Q_heat [W]/1

== system Vehicle_cl/Vehicle/Thermal System/Engine Thermal Model/EGR Loop ==
  T_cool_ENG_in [K] : Inport
  Add : Sum
  Constant : Constant  Value=TSTAT.tau  VectorParams1D=off
  Divide : Product  Inputs=*//
  Divide1 : Product  Inputs=*/
  Gain : Gain  Gain=2
  Integrator : Integrator  InitialCondition=ETM.T_init
  Sum : Sum  Inputs=+-
  T_cool_EGR_out [K] : Outport  VectorParamsAs1DForOutWhenUnconnected=off
  wires:
  Divide/1 -> Add/2
  [m_dot_EGR] -> Divide/2
  [cp_cool] -> Divide/3
  T_cool_ENG_in [K]/1 -> Add/1
  [Q_dot_EGR] -> Gain/1
  Gain/1 -> Divide/1
  Add/1 -> Sum/1
  Divide1/1 -> Integrator/1
  Sum/1 -> Divide1/1
  Constant/1 -> Divide1/2
  Integrator/1 -> Sum/2, T_cool_EGR_out [K]/1

== system Vehicle_cl/Vehicle/Thermal System/Engine Thermal Model/Engine Thermal Model (Single Mass) ==
  T_cool_ENG_in [K] : Inport
  Mass 1: Block : Subsystem
  T_cool_ENG_out [K] : Outport  VectorParamsAs1DForOutWhenUnconnected=off
  tag scope: T_cool_out=scoped
  wires:
  Mass 1: Block/1(T1 [K]) -> T_cool_ENG_out [K]/1, [T_cool_out]
  [Q_dot_heat] -> Mass 1: Block/1(Q_dot_heat [W])
  [Q_dot_fr] -> Mass 1: Block/2(Q_dot_fr [W])
  [m_dot_ENG] -> Mass 1: Block/4(m_dot_cool [kg/s])
  T_cool_ENG_in [K]/1 -> Mass 1: Block/3(T_cool_in [K])

== system Vehicle_cl/Vehicle/Thermal System/Engine Thermal Model/Mixing EGR and Engine ==
  T_cool_ENG_out [K] : Inport
  T_cool_EGR_out [K] : Inport  Port=2
  Add : Sum
  Add1 : Sum
  Product1 : Product
  Product2 : Product
  Product3 : Product  Inputs=*/
  T_cool_RAD in [K] : Outport  VectorParamsAs1DForOutWhenUnconnected=off
  wires:
  [m_dot_EGR] -> Add1/1
  Add1/1 -> Product3/2
  Product2/1 -> Add/1
  T_cool_EGR_out [K]/1 -> Product1/1
  [m_dot_ENG] -> Product2/2
  Product1/1 -> Add/2
  T_cool_ENG_out [K]/1 -> Product2/1
  [m_dot_ENG] -> Add1/2
  Add/1 -> Product3/1
  [m_dot_EGR] -> Product1/2
  Product3/1 -> T_cool_RAD in [K]/1

== system Vehicle_cl/Vehicle/Thermal System/Engine Thermal Model/Mixing at Pump Inlet  ==
  T_cool_RAD_out [K] : Inport
  T_cool_RAD_in [K] : Inport  Port=2
  Add2 : Sum
  Add3 : Sum
  Product4 : Product
  Product5 : Product
  Product6 : Product  Inputs=*/
  Transfer Fcn (with initial outputs) : simulink_extras/Additional Linear/Transfer Fcn (with initial outputs)  N=[1]  D=[ .11 1]  Y0=ETM.T_init  U0=0
  T_cool_ENG_in [K] : Outport  VectorParamsAs1DForOutWhenUnconnected=off
  wires:
  T_cool_RAD_out [K]/1 -> Product4/1
  Product4/1 -> Add2/1
  Product6/1 -> Transfer Fcn (with initial outputs)/1
  Add2/1 -> Product6/1
  [m_dot_BYPASS] -> Add3/2
  [m_dot_RAD] -> Add3/1
  Add3/1 -> Product6/2
  T_cool_RAD_in [K]/1 -> Product5/1  "T_cool_bypass"
  Product5/1 -> Add2/2
  [m_dot_RAD] -> Product4/2
  [m_dot_BYPASS] -> Product5/2
  Transfer Fcn (with initial outputs)/1 -> T_cool_ENG_in [K]/1

== system Vehicle_cl/Vehicle/Thermal System/Engine Thermal Model/Reduced Radiator Thermal Model (1 Node - 1 Mass) ==
  T_cool_RAD_in [K] : Inport
  m_dot_RAD [kg/s] : Inport  Port=2
  T_air [K] : Inport  Port=3
  V_face [m/s] : Inport  Port=4
  Divide3 : Product  Inputs=***
  Radiator Thermal Model : Subsystem
  Sum3 : Sum  Inputs=+-
  T_cool_RAD_out [K] : Outport  VectorParamsAs1DForOutWhenUnconnected=off
  Q_dot_RAD [W] : Outport  Port=2  VectorParamsAs1DForOutWhenUnconnected=off
  wires:
  m_dot_RAD [kg/s]/1 -> Radiator Thermal Model/1(m_dot_RAD [kg/s]), Divide3/1
  V_face [m/s]/1 -> Radiator Thermal Model/3(Vf)
  Divide3/1 -> Q_dot_RAD [W]/1
  Radiator Thermal Model/1(Tc) -> Sum3/2, T_cool_RAD_out [K]/1
  T_air [K]/1 -> Radiator Thermal Model/2(T_air)
  T_cool_RAD_in [K]/1 -> Radiator Thermal Model/4("T_RAD_in [K] "), Sum3/1
  [cp_cool] -> Divide3/2
  Sum3/1 -> Divide3/3

== system Vehicle_cl/Vehicle/Vehicle Road Load/Subsystem/Disengaged ==
  RPM init : Inport
  T_eng : Inport  Port=2
  Enable : EnablePort  StatesWhenEnabling=reset
  Gain1 : Gain  Gain=1/VEH.inertiaCrank
  Integrator : Integrator  InitialConditionSource=external
  Out1 : Outport  InitialOutput=ICE.Nmin  VectorParamsAs1DForOutWhenUnconnected=off
  wires:
  Integrator/1 -> Out1/1
  T_eng/1 -> Gain1/1
  Gain1/1 -> Integrator/1
  RPM init/1 -> Integrator/2

== system Vehicle_cl/Vehicle/Vehicle Road Load/Subsystem/Engaged ==
  Vehicle Speed [m/s] : Inport
  drive ratio : Inport  Port=2
  Enable : EnablePort  StatesWhenEnabling=reset
  Divide1 : Product  Inputs=**
  Gain2 : Gain  Gain=30/pi
  Gain3 : Gain  Gain=1/VEH.tireRad
  Out1 : Outport  InitialOutput=ICE.Nmin  VectorParamsAs1DForOutWhenUnconnected=off
  wires:
  Gain2/1 -> Divide1/1  "tire rpm"
  Gain3/1 -> Gain2/1
  drive ratio/1 -> Divide1/2
  Vehicle Speed [m/s]/1 -> Gain3/1
  Divide1/1 -> Out1/1

== system Vehicle_cl/Vehicle/Thermal System/Engine Thermal Model/Engine Thermal Model (Single Mass)/Mass 1: Block ==
  note: Energy Balance
  Q_dot_heat [W] : Inport
  Q_dot_fr [W] : Inport  Port=2
  T_cool_in [K] : Inport  Port=3
  m_dot_cool [kg/s] : Inport  Port=4
  Gain : Gain  Gain=1/ETM.C1
  Integrator : Integrator  InitialCondition=ETM.T_init
  Product1 : Product  Inputs=3
  Sum3 : Sum  Inputs=++-
  Sum4 : Sum  Inputs=+-
  T1 [K] : Outport  VectorParamsAs1DForOutWhenUnconnected=off
  wires:
  Q_dot_fr [W]/1 -> Sum3/2  "Friction Heat to Block (W)"
  Sum3/1 -> Gain/1
  Q_dot_heat [W]/1 -> Sum3/1  "Engine Heat Rejection (W)"
  Gain/1 -> Integrator/1
  Integrator/1 -> T1 [K]/1
  T_cool_in [K]/1 -> Sum4/2
  [T_cool_out] -> Sum4/1
  [cp_cool] -> Product1/2
  m_dot_cool [kg/s]/1 -> Product1/3
  Sum4/1 -> Product1/1
  Product1/1 -> Sum3/3

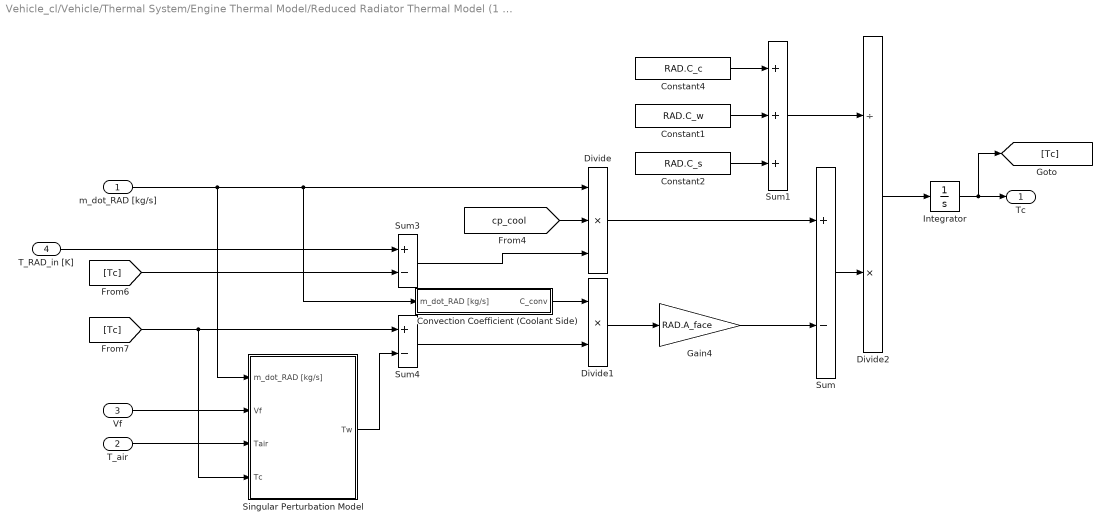
== system Vehicle_cl/Vehicle/Thermal System/Engine Thermal Model/Reduced Radiator Thermal Model (1 Node - 1 Mass)/Radiator Thermal Model ==
  m_dot_RAD [kg/s] : Inport
  T_air : Inport  Port=2
  Vf : Inport  Port=3
  "T_RAD_in [K] " : Inport  Port=4
  Constant1 : Constant  Value=RAD.C_w
  Constant2 : Constant  Value=RAD.C_s
  Constant4 : Constant  Value=RAD.C_c
  Convection Coefficient (Coolant Side) : Subsystem
  Divide : Product  Inputs=***
  Divide1 : Product  Inputs=**
  Divide2 : Product  Inputs=/*
  Gain4 : Gain  Gain=RAD.A_face
  Integrator : Integrator  InitialCondition=RAD.T_init
  Singular Perturbation Model : Subsystem
  Sum : Sum  Inputs=+-
  Sum1 : Sum  Inputs=+++
  Sum3 : Sum  Inputs=+-
  Sum4 : Sum  Inputs=+-
  Tc : Outport  VectorParamsAs1DForOutWhenUnconnected=off
  wires:
  Singular Perturbation Model/1(Tw) -> Sum4/2
  T_air/1 -> Singular Perturbation Model/3(Tair)
  Sum4/1 -> Divide1/2
  Vf/1 -> Singular Perturbation Model/2(Vf)
  Divide1/1 -> Gain4/1
  Gain4/1 -> Sum/2
  Divide/1 -> Sum/1
  m_dot_RAD [kg/s]/1 -> Singular Perturbation Model/1(m_dot_RAD [kg/s]), Convection Coefficient (Coolant Side)/1(m_dot_RAD [kg/s]), Divide/1
  Sum/1 -> Divide2/2
  Divide2/1 -> Integrator/1
  Integrator/1 -> [Tc], Tc/1
  Convection Coefficient (Coolant Side)/1(C_conv) -> Divide1/1
  [cp_cool] -> Divide/2
  Sum3/1 -> Divide/3
  Constant2/1 -> Sum1/3
  Constant1/1 -> Sum1/2
  Constant4/1 -> Sum1/1
  "T_RAD_in [K] "/1 -> Sum3/1
  [Tc] -> Sum3/2
  [Tc] -> Singular Perturbation Model/4(Tc), Sum4/1
  Sum1/1 -> Divide2/1

== system Vehicle_cl/Vehicle/Thermal System/Engine Thermal Model/Reduced Radiator Thermal Model (1 Node - 1 Mass)/Radiator Thermal Model/Convection Coefficient (Coolant Side) ==
  m_dot_RAD [kg/s] : Inport
  Constant : Constant  Value=RAD.C_convMIN
  Constant1 : Constant  Value=RAD.beta
  Constant3 : Constant  Value=RAD.C_f
  Constant4 : Constant  Value=RAD.C3
  Divide4 : Product  Inputs=**/
  Math Function2 : Math  Operator=pow  SignedPower=on  SaturateOnIntegerOverflow=on
  Switch : Switch  Criteria=u2 > Threshold  Threshold=0.01
  m_dot_RAD [kg/s]1 : InportShadow
  C_conv : Outport  VectorParamsAs1DForOutWhenUnconnected=off
  wires:
  Constant3/1 -> Divide4/1  "Cf"
  Constant1/1 -> Math Function2/2
  m_dot_RAD [kg/s]/1 -> Math Function2/1
  Math Function2/1 -> Divide4/2
  Divide4/1 -> Switch/1
  Constant/1 -> Switch/3
  Switch/1 -> C_conv/1
  m_dot_RAD [kg/s]1/1 -> Switch/2
  Constant4/1 -> Divide4/3

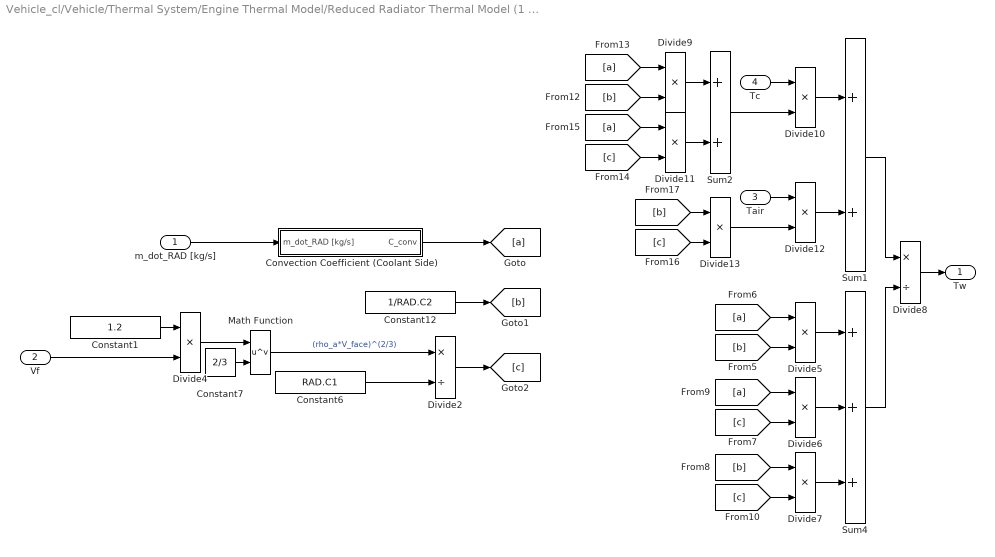
== system Vehicle_cl/Vehicle/Thermal System/Engine Thermal Model/Reduced Radiator Thermal Model (1 Node - 1 Mass)/Radiator Thermal Model/Singular Perturbation Model ==
  m_dot_RAD [kg/s] : Inport
  Vf : Inport  Port=2
  Tair : Inport  Port=3
  Tc : Inport  Port=4
  Constant1 : Constant  Value=1.2
  Constant12 : Constant  Value=1/RAD.C2
  Constant6 : Constant  Value=RAD.C1
  Constant7 : Constant  Value=2/3
  Convection Coefficient (Coolant Side) : Subsystem
  Divide{4..7,9..13} (9 alike) : Product  Inputs=**
  Divide2 : Product  Inputs=*/
  Divide8 : Product  Inputs=*/
  Math Function : Math  Operator=pow  SignedPower=on  SaturateOnIntegerOverflow=on
  Sum1 : Sum
  Sum2 : Sum
  Sum4 : Sum  Inputs=+++
  Tw : Outport  VectorParamsAs1DForOutWhenUnconnected=off
  wires:
  Divide8/1 -> Tw/1
  Vf/1 -> Divide4/2
  Constant1/1 -> Divide4/1
  Constant6/1 -> Divide2/2
  Math Function/1 -> Divide2/1  "(rho_a*V_face)^(2/3)"
  Constant7/1 -> Math Function/2
  Divide4/1 -> Math Function/1
  [a] -> Divide5/1
  [b] -> Divide5/2
  [a] -> Divide6/1
  [c] -> Divide6/2
  [b] -> Divide7/1
  [c] -> Divide7/2
  Divide5/1 -> Sum4/1
  Divide6/1 -> Sum4/2
  Divide7/1 -> Sum4/3
  Sum4/1 -> Divide8/2
  Sum1/1 -> Divide8/1
  Divide12/1 -> Sum1/2
  [b] -> Divide13/1
  [c] -> Divide13/2
  Divide13/1 -> Divide12/2
  [a] -> Divide9/1
  [b] -> Divide9/2
  Tair/1 -> Divide12/1
  Divide10/1 -> Sum1/1
  Tc/1 -> Divide10/1
  [a] -> Divide11/1
  [c] -> Divide11/2
  Divide9/1 -> Sum2/1
  Divide11/1 -> Sum2/2
  Sum2/1 -> Divide10/2
  m_dot_RAD [kg/s]/1 -> Convection Coefficient (Coolant Side)/1(m_dot_RAD [kg/s])
  Constant12/1 -> [b]
  Convection Coefficient (Coolant Side)/1(C_conv) -> [a]
  Divide2/1 -> [c]

== system Vehicle_cl/Vehicle/Thermal System/Engine Thermal Model/Reduced Radiator Thermal Model (1 Node - 1 Mass)/Radiator Thermal Model/Singular Perturbation Model/Convection Coefficient (Coolant Side) ==
  m_dot_RAD [kg/s] : Inport
  Constant : Constant  Value=RAD.C_convMIN
  Constant1 : Constant  Value=RAD.beta
  Constant3 : Constant  Value=RAD.C_f
  Constant4 : Constant  Value=RAD.C3
  Divide4 : Product  Inputs=**/
  Math Function2 : Math  Operator=pow  SignedPower=on  SaturateOnIntegerOverflow=on
  Switch : Switch  Criteria=u2 > Threshold  Threshold=0.01
  m_dot_RAD [kg/s]1 : InportShadow
  C_conv : Outport  VectorParamsAs1DForOutWhenUnconnected=off
  wires:
  Constant3/1 -> Divide4/1  "Cf"
  Constant1/1 -> Math Function2/2
  m_dot_RAD [kg/s]/1 -> Math Function2/1
  Math Function2/1 -> Divide4/2
  Divide4/1 -> Switch/1
  Constant/1 -> Switch/3
  Switch/1 -> C_conv/1
  m_dot_RAD [kg/s]1/1 -> Switch/2
  Constant4/1 -> Divide4/3
